simulink model "data_filtering"  (R2019b)
settings: Solver=FixedStepAuto  StartTime=0.0  StopTime=60  FixedStep=0.001  RelTol=1e-3
libraries: dsparch4 x8
settings Model: Creator=Alexander  LastModifiedBy=Alexander

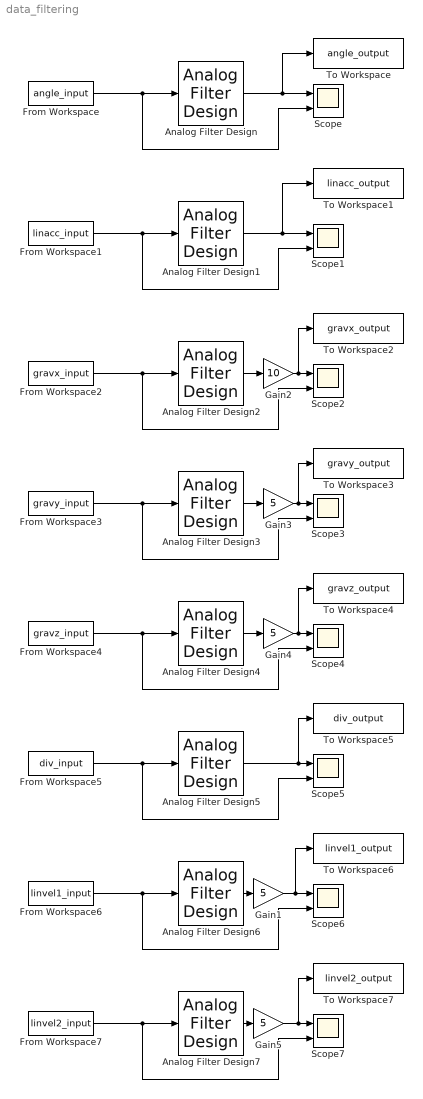
== system data_filtering ==
  Analog Filter Design : dsparch4/Analog Filter Design  method=Butterworth  filttype=Bandpass  N=8  Wlo=0.1*2*pi  Whi=6*2*pi  Rp=2  Rs=40
  Analog Filter Design1 : dsparch4/Analog Filter Design  method=Butterworth  filttype=Lowpass  N=8  Wlo=4*2*pi  Whi=5*2*pi  Rp=2  Rs=40
  Analog Filter Design2 : dsparch4/Analog Filter Design  method=Butterworth  filttype=Lowpass  N=8  Wlo=5*2*pi  Whi=5*2*pi  Rp=2  Rs=40
  Analog Filter Design3 : dsparch4/Analog Filter Design  method=Butterworth  filttype=Lowpass  N=8  Wlo=3*2*pi  Whi=5*2*pi  Rp=2  Rs=40
  Analog Filter Design4 : dsparch4/Analog Filter Design  method=Butterworth  filttype=Lowpass  N=8  Wlo=4*2*pi  Whi=5*2*pi  Rp=2  Rs=40
  Analog Filter Design5 : dsparch4/Analog Filter Design  method=Butterworth  filttype=Lowpass  N=50  Wlo=3.5*2*pi  Whi=3*2*pi  Rp=2  Rs=40
  Analog Filter Design6 : dsparch4/Analog Filter Design  method=Butterworth  filttype=Highpass  N=4  Wlo=0.2*2*pi  Whi=3*2*pi  Rp=2  Rs=40
  Analog Filter Design7 : dsparch4/Analog Filter Design  method=Butterworth  filttype=Highpass  N=4  Wlo=0.2*2*pi  Whi=3*2*pi  Rp=2  Rs=40
  From Workspace : FromWorkspace  VariableName=angle_input  SampleTime=0
  From Workspace1 : FromWorkspace  VariableName=linacc_input  SampleTime=0
  From Workspace2 : FromWorkspace  VariableName=gravx_input  SampleTime=0
  From Workspace3 : FromWorkspace  VariableName=gravy_input  SampleTime=0
  From Workspace4 : FromWorkspace  VariableName=gravz_input  SampleTime=0
  From Workspace5 : FromWorkspace  VariableName=div_input  SampleTime=0
  From Workspace6 : FromWorkspace  VariableName=linvel1_input  SampleTime=0
  From Workspace7 : FromWorkspace  VariableName=linvel2_input  SampleTime=0
  Gain{1,3..5} (4 alike) : Gain  Gain=5
  Gain2 : Gain  Gain=10
  Scope{,1..7} (8 alike) : Scope  NumInputPorts=2
  To Workspace : ToWorkspace  VariableName=angle_output  SaveFormat=Structure With Time  SampleTime=-1
  To Workspace1 : ToWorkspace  VariableName=linacc_output  SaveFormat=Structure With Time  SampleTime=-1
  To Workspace2 : ToWorkspace  VariableName=gravx_output  SaveFormat=Structure With Time  SampleTime=-1
  To Workspace3 : ToWorkspace  VariableName=gravy_output  SaveFormat=Structure With Time  SampleTime=-1
  To Workspace4 : ToWorkspace  VariableName=gravz_output  SaveFormat=Structure With Time  SampleTime=-1
  To Workspace5 : ToWorkspace  VariableName=div_output  SaveFormat=Structure With Time  SampleTime=-1
  To Workspace6 : ToWorkspace  VariableName=linvel1_output  SaveFormat=Structure With Time  SampleTime=-1
  To Workspace7 : ToWorkspace  VariableName=linvel2_output  SaveFormat=Structure With Time  SampleTime=-1
  wires:
  From Workspace/1 -> Scope/2, Analog Filter Design/1
  Analog Filter Design/1 -> To Workspace/1, Scope/1
  Analog Filter Design1/1 -> To Workspace1/1, Scope1/1
  From Workspace1/1 -> Scope1/2, Analog Filter Design1/1
  Analog Filter Design2/1 -> Gain2/1
  Gain2/1 -> To Workspace2/1, Scope2/1
  From Workspace2/1 -> Scope2/2, Analog Filter Design2/1
  Analog Filter Design3/1 -> Gain3/1
  Gain3/1 -> To Workspace3/1, Scope3/1
  From Workspace3/1 -> Scope3/2, Analog Filter Design3/1
  Analog Filter Design4/1 -> Gain4/1
  Gain4/1 -> To Workspace4/1, Scope4/1
  From Workspace4/1 -> Scope4/2, Analog Filter Design4/1
  From Workspace5/1 -> Scope5/2, Analog Filter Design5/1
  Analog Filter Design5/1 -> To Workspace5/1, Scope5/1
  From Workspace6/1 -> Scope6/2, Analog Filter Design6/1
  From Workspace7/1 -> Scope7/2, Analog Filter Design7/1
  Analog Filter Design6/1 -> Gain1/1
  Gain1/1 -> To Workspace6/1, Scope6/1
  Analog Filter Design7/1 -> Gain5/1
  Gain5/1 -> To Workspace7/1, Scope7/1
